simulink model "DCM_Ideal_Supply"  (R2025a)
settings: Solver=ode5  StartTime=0.0  StopTime=6  FixedStep=dt  RelTol=1e-3  EnableMultiTasking=on
values from neighbouring files (symbols this model uses):
  a1 = -1.122    [Experiment_1_DCM_Parameter.m]
  a2 = 2.553    [Experiment_1_DCM_Parameter.m]
  a3 = -0.759    [Experiment_1_DCM_Parameter.m]
  C_M = 0.96    [Experiment_1_DCM_Parameter.m]
  dt = 1e-5    (= 1e-05)    [Experiment_1_DCM_Parameter.m]
  I_EN = 0.1    [Experiment_1_DCM_Parameter.m]
  L_A = 374e-3    (= 0.374)    [Experiment_1_DCM_Parameter.m]
  M_MN = 0.955    [Experiment_1_DCM_Parameter.m]
  R_A = 22    [Experiment_1_DCM_Parameter.m]
  R_E = 2200    [Experiment_1_DCM_Parameter.m]
  Theta_M = 0.0013    [Experiment_1_DCM_Parameter.m]
  U_AN = 220    [Experiment_1_DCM_Parameter.m]
  U_EN = 220    [Experiment_1_DCM_Parameter.m]
libraries: simulink x2
settings Model: Creator=BinLi  LastModifiedBy=lucaslee
settings SolverCC: AlgebraicLoopSolver=TrustRegion
settings DataIOCC: LimitDataPoints=on  SaveFormat=Array  SignalLoggingSaveFormat=ModelDataLogs  ReturnWorkspaceOutputs=off
settings OptimizationCC: ExpressionDepthLimit=2147483647.0  LifeSpan=inf
settings DebuggingCC: UnderspecifiedInitializationDetection=Classic  MergeDetectMultiDrivingBlocksExec=none  SolverPrmCheckMsg=warning  FcnCallInpInsideContextMsg=warning  UnconnectedInputMsg=warning  UnconnectedOutputMsg=warning  UnconnectedLineMsg=warning  StateNameClashWarn=warning  SFUnexpectedBacktrackingDiag=warning  SFNoUnconditionalDefaultTransitionDiag=warning  SFExecutionAtInitializationDiag=none  ArithmeticOperatorsInVariantConditions=warning
settings HardwareCC: ProdBitPerPointer=32.0  ProdBitPerSizeT=32.0  ProdBitPerPtrDiffT=32.0  ProdLargestAtomicFloat=None  ProdIntDivRoundTo=Undefined  ProdEndianess=Unspecified  ProdWordSize=32.0  ProdHWDeviceType=32-bit Generic
settings ModelReferenceCC: EnableRefExpFcnMdlSchedulingChecks=on  PropagateSignalLabelsOutOfModel=off
settings SFSimCC: SimUseLocalCustomCode=off  CustomCodeUndefinedFunction=UseInterfaceOnly
settings RTWCC: RTWUseLocalCustomCode=off  GPUComputeCapability=3.5
settings CodeAppCC: StateflowObjectComments=on
settings GRTTargetCC: TargetLangStandard=C89/C90 (ANSI)  CombineOutputUpdateFcns=off  GRTInterface=on
settings ConfigComp: CovMetricSettings=dw  CovSaveCumulativeToWorkspaceVar=on  CovSaveSingleToWorkspaceVar=on  CovExternalEMLEnable=off  CovSFcnEnable=off

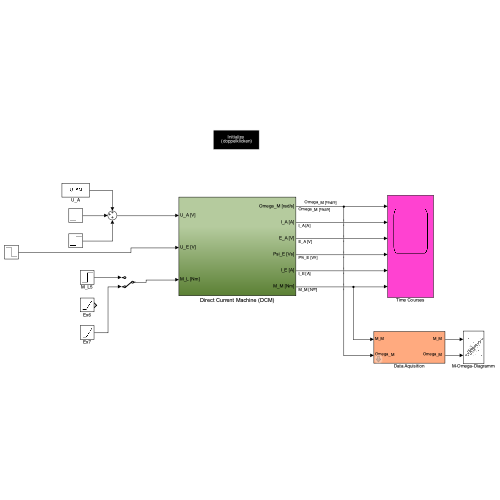
[thumbnail: Simulink's stored preview of the top-level diagram]
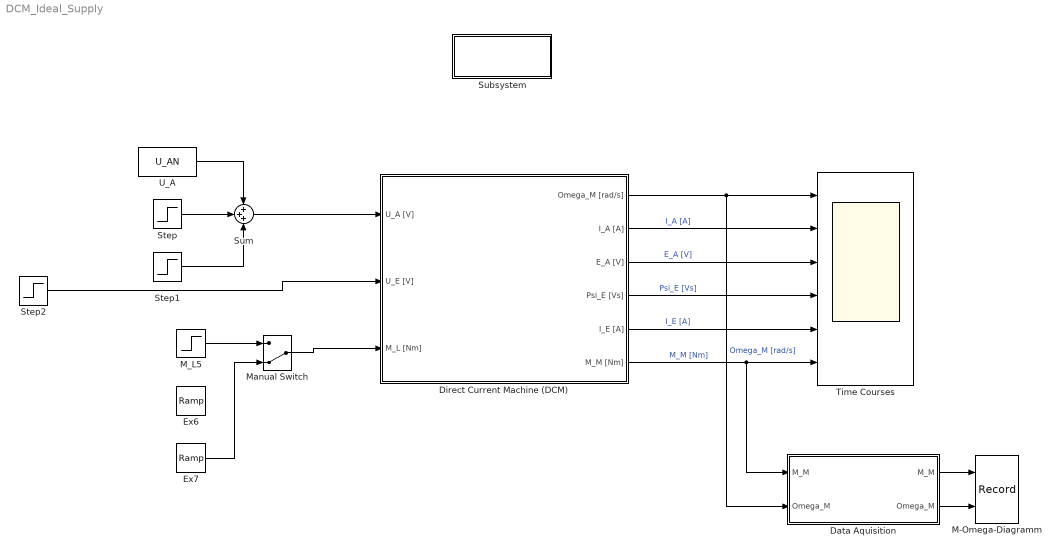
== system DCM_Ideal_Supply ==
  Data Aquisition : Subsystem  mask{downsampling=100}
  Direct Current Machine (DCM) : Subsystem
  Ex6 : simulink/Sources/Ramp  slope=M_MN*6  start=0  InitialOutput=-M_MN
  Ex7 : simulink/Sources/Ramp  slope=M_MN  start=0.2  InitialOutput=0
  M-Omega-Diagramm : Record  NumPorts=2.0  FileSettingsInternal="{\"entries\":[{\"content\":{\"excelSettings\":{\"content\":{},\"type\":\"Streamout.ExcelSettings\"},\"parquetSettings\":{\"content\":{},\"type\":\"Streamout.ParquetSettings\"}},\"type\":\"Streamout.FileSettingStorage\",\"uuid\":\"\"}],\"packageUris\":[\"http:\\/\\/schema.mathworks.com\\/mf0\\/streamout_blocks\\/R2020a\"],\"version\":\"1.0\"}"  FrameSettings=[0, 0]  Layout=[1 1]  SignalsInternal="{\"entries\":[{\"content\":{\"signals\":[{\"content\":{\"blockPath\":[],\"dimensions\":[1],\"domain\":\"\",\"lineColor\":\"#a2142f\",\"plots\":[ 1 ],\"port\":1,\"signalID\":1,\"signalName\":\"Data Aquisition:1\"},\"type\":\"RecordBlkView.Signal\",\"uuid\":\"\"},{\"content\":{\"blockPath\":[],\"dimensions\":[1],\"domain\":\"\",\"lineColor\":\"#139fff\",\"plots\":[ 1 ],\"port\":2,\"signalID\":2,\"signalName\":\"Data Aquisition:2\"},\"type\":\"RecordBlkView.Signal\",\"uuid\":\"\"}]},\"type\":\"RecordBlkView.InputSignals\",\"uuid\":\"\"}],\"packageUris\":[\"http:\\/\\/schema.mathworks.com\\/mf0\\/streamout_blocks\\/R2020a\"],\"version\":\"1.0\"}"  VisualizationBindings="{\"xyplotplugin\":{\"info\":[{\"series\":[{\"bindingParametersList\":[{\"parameter\":\"X-Axis\",\"signalID\":1,\"signalName\":\"Data Aquisition:1\"},{\"parameter\":\"Y-Axis\",\"signalID\":2,\"signalName\":\"Data Aquisition:2\"}],\"seriesID\":0}],\"subplotID\":1}]}}"  CompatibilityTag=XY  st=-1
  M_L5 : Step  After=M_MN  SampleTime=0
  Manual Switch : ManualSwitch  CurrentSetting=0
  Step : Step  Time=3  After=0  SampleTime=0
  Step1 : Step  Time=5  After=0  SampleTime=0
  Step2 : Step  Time=3  Before=U_EN  After=0.5*U_EN  SampleTime=0
  Subsystem : Subsystem
      settings: OpenFcn=Experiment_1_DCM_Parameter
      mask Display: disp('Initialize\n (doppelklicken)')
  Sum : Sum  Inputs=+++
  Time Courses : Scope  NumInputPorts=6
      settings: TimeSpan=0.1  ActiveDisplayYMinimum=-26.176467394341685  ActiveDisplayYMaximum=235.58820654907524
  U_A : Constant  Value=U_AN
  wires:
  Direct Current Machine (DCM)/1(Omega_M [rad/s]) -> Data Aquisition/2(Omega_M), Time Courses/1  "Omega_M [rad/s]"
  Direct Current Machine (DCM)/2(I_A [A]) -> Time Courses/2  "I_A [A]"
  Direct Current Machine (DCM)/5(I_E [A]) -> Time Courses/5  "I_E [A]"
  Direct Current Machine (DCM)/6(M_M [Nm]) -> Time Courses/6, Data Aquisition/1(M_M)  "M_M [Nm]"
  Direct Current Machine (DCM)/3(E_A [V]) -> Time Courses/3  "E_A [V]"
  Direct Current Machine (DCM)/4(Psi_E [Vs]) -> Time Courses/4  "Psi_E [Vs]"
  Data Aquisition/1("M_M ") -> M-Omega-Diagramm/1
  Data Aquisition/2("Omega_M ") -> M-Omega-Diagramm/2
  Step2/1 -> Direct Current Machine (DCM)/2(U_E [V])
  M_L5/1 -> Manual Switch/1
  Manual Switch/1 -> Direct Current Machine (DCM)/3(M_L [Nm])
  Sum/1 -> Direct Current Machine (DCM)/1(U_A [V])
  Ex7/1 -> Manual Switch/2
  U_A/1 -> Sum/1
  Step/1 -> Sum/2
  Step1/1 -> Sum/3

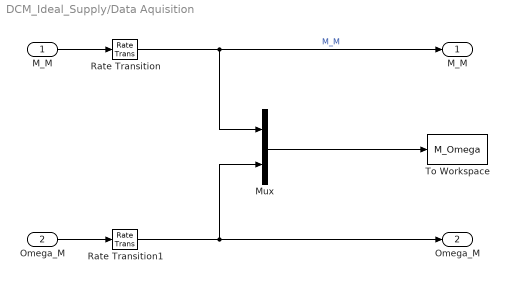
== system DCM_Ideal_Supply/Data Aquisition ==
  M_M : Inport
  Omega_M : Inport  Port=2
  Mux : Mux  Inputs=2
  Rate Transition : RateTransition  OutPortSampleTime=downsampling*dt
  Rate Transition1 : RateTransition  OutPortSampleTime=downsampling*dt
  To Workspace : ToWorkspace  VariableName=M_Omega  SaveFormat=Structure  SampleTime=-1
  "M_M " : Outport
  "Omega_M " : Outport  Port=2
  wires:
  Mux/1 -> To Workspace/1
  Rate Transition/1 -> Mux/1, "M_M "/1  "M_M"
  Rate Transition1/1 -> Mux/2, "Omega_M "/1
  Omega_M/1 -> Rate Transition1/1
  M_M/1 -> Rate Transition/1

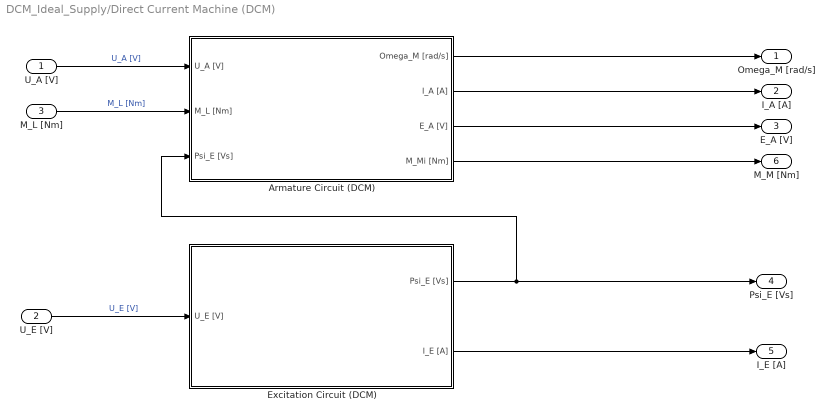
== system DCM_Ideal_Supply/Direct Current Machine (DCM) ==
  U_A [V] : Inport
  U_E [V] : Inport  Port=2
  M_L [Nm] : Inport  Port=3
  Armature Circuit (DCM) : Subsystem
  Excitation Circuit (DCM) : Subsystem
  Omega_M [rad/s] : Outport  InitialOutput=0
  I_A [A] : Outport  Port=2  InitialOutput=0
  E_A [V] : Outport  Port=3  InitialOutput=0
  Psi_E [Vs] : Outport  Port=4  InitialOutput=0
  I_E [A] : Outport  Port=5  InitialOutput=0
  M_M [Nm] : Outport  Port=6  InitialOutput=0
  wires:
  Armature Circuit (DCM)/4(M_Mi [Nm]) -> M_M [Nm]/1
  Excitation Circuit (DCM)/2(I_E [A]) -> I_E [A]/1
  Armature Circuit (DCM)/3(E_A [V]) -> E_A [V]/1
  Armature Circuit (DCM)/2(I_A [A]) -> I_A [A]/1
  U_E [V]/1 -> Excitation Circuit (DCM)/1(U_E [V])  "U_E [V]"
  Armature Circuit (DCM)/1(Omega_M [rad/s]) -> Omega_M [rad/s]/1
  Excitation Circuit (DCM)/1(Psi_E [Vs]) -> Psi_E [Vs]/1, Armature Circuit (DCM)/3(Psi_E [Vs])
  M_L [Nm]/1 -> Armature Circuit (DCM)/2(M_L [Nm])  "M_L [Nm]"
  U_A [V]/1 -> Armature Circuit (DCM)/1(U_A [V])  "U_A [V]"

== system DCM_Ideal_Supply/Subsystem ==

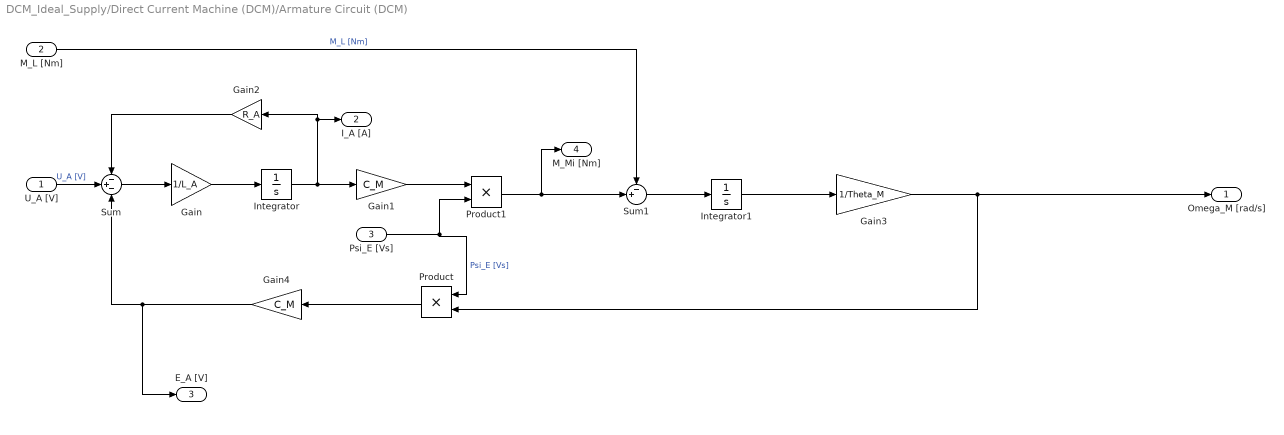
== system DCM_Ideal_Supply/Direct Current Machine (DCM)/Armature Circuit (DCM) ==
  U_A [V] : Inport
  M_L [Nm] : Inport  Port=2
  Psi_E [Vs] : Inport  Port=3
  Gain : Gain  Gain=1/L_A
  Gain1 : Gain  Gain=C_M
  Gain2 : Gain  Gain=R_A
  Gain3 : Gain  Gain=1/Theta_M
  Gain4 : Gain  Gain=C_M
  Integrator : Integrator
  Integrator1 : Integrator
  Product : Product
  Product1 : Product
  Sum : Sum  Inputs=-+-
  Sum1 : Sum  Inputs=-+|
  Omega_M [rad/s] : Outport  InitialOutput=0
  I_A [A] : Outport  Port=2  InitialOutput=0
  E_A [V] : Outport  Port=3  InitialOutput=0
  M_Mi [Nm] : Outport  Port=4  InitialOutput=0
  wires:
  Sum/1 -> Gain/1
  Gain/1 -> Integrator/1
  Gain1/1 -> Product1/1
  Product1/1 -> M_Mi [Nm]/1, Sum1/2
  M_L [Nm]/1 -> Sum1/1  "M_L [Nm]"
  Integrator/1 -> I_A [A]/1, Gain2/1, Gain1/1
  Gain2/1 -> Sum/1
  U_A [V]/1 -> Sum/2  "U_A [V]"
  Psi_E [Vs]/1 -> Product1/2, Product/1  "Psi_E [Vs]"
  Sum1/1 -> Integrator1/1
  Integrator1/1 -> Gain3/1
  Gain3/1 -> Product/2, Omega_M [rad/s]/1
  Product/1 -> Gain4/1
  Gain4/1 -> E_A [V]/1, Sum/3

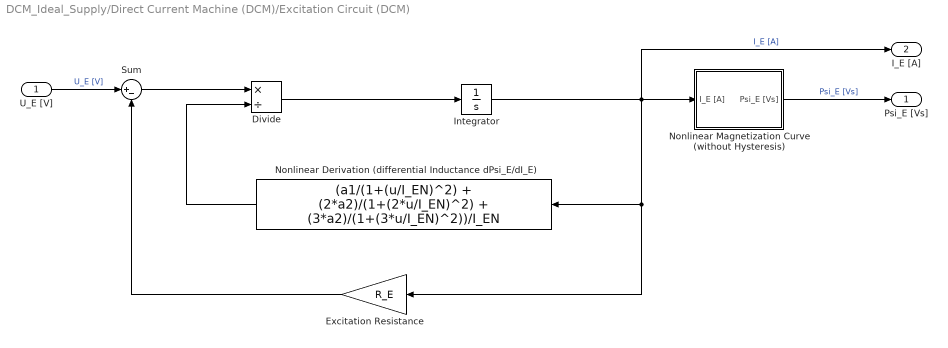
== system DCM_Ideal_Supply/Direct Current Machine (DCM)/Excitation Circuit (DCM) ==
  U_E [V] : Inport
  Divide : Product  Inputs=*/
  Excitation Resistance : Gain  Gain=R_E
  Integrator : Integrator
  Nonlinear Derivation (differential Inductance dPsi_E/dI_E) : Fcn  Expr=(a1/(1+(u/I_EN)^2) + (2*a2)/(1+(2*u/I_EN)^2) + (3*a2)/(1+(3*u/I_EN)^2))/I_EN
  Nonlinear Magnetization Curve (without Hysteresis) : Subsystem
      mask Display:
      | plot([-5:0.1:5], 2/pi*atan([-5:0.1:5]./1.5) + 0.05.*[-5:0.1:5]);
      | plot([0 0],[-1.25 1.25]);
      | plot([-5 5],[0 0]);
  Sum : Sum  Inputs=|+-  InputSameDT=on  SaturateOnIntegerOverflow=on  OutDataTypeStr=Inherit: Same as first input
  Psi_E [Vs] : Outport  InitialOutput=0
  I_E [A] : Outport  Port=2  InitialOutput=0
  wires:
  Nonlinear Magnetization Curve (without Hysteresis)/1(Psi_E [Vs]) -> Psi_E [Vs]/1  "Psi_E [Vs]"
  U_E [V]/1 -> Sum/1  "U_E [V]"
  Excitation Resistance/1 -> Sum/2
  Sum/1 -> Divide/1
  Nonlinear Derivation (differential Inductance dPsi_E/dI_E)/1 -> Divide/2
  Integrator/1 -> I_E [A]/1, Nonlinear Magnetization Curve (without Hysteresis)/1(I_E [A]), Excitation Resistance/1, Nonlinear Derivation (differential Inductance dPsi_E/dI_E)/1  "I_E [A]"
  Divide/1 -> Integrator/1

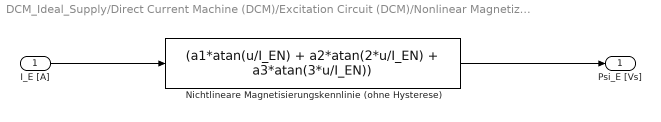
== system DCM_Ideal_Supply/Direct Current Machine (DCM)/Excitation Circuit (DCM)/Nonlinear Magnetization Curve (without Hysteresis) ==
  I_E [A] : Inport
  Nichtlineare Magnetisierungskennlinie (ohne Hysterese) : Fcn  Expr=(a1*atan(u/I_EN) + a2*atan(2*u/I_EN) + a3*atan(3*u/I_EN))
  Psi_E [Vs] : Outport
  wires:
  I_E [A]/1 -> Nichtlineare Magnetisierungskennlinie (ohne Hysterese)/1
  Nichtlineare Magnetisierungskennlinie (ohne Hysterese)/1 -> Psi_E [Vs]/1
